simulink model "fft01c"  (R2023a)
settings: Solver=VariableStepAuto  StartTime=0.0  StopTime=10.0  RelTol=1e-3
libraries: dspsrcs4 x3, dspxfrm3 x2
settings Model: Creator=2361266  LastModifiedBy=2361266

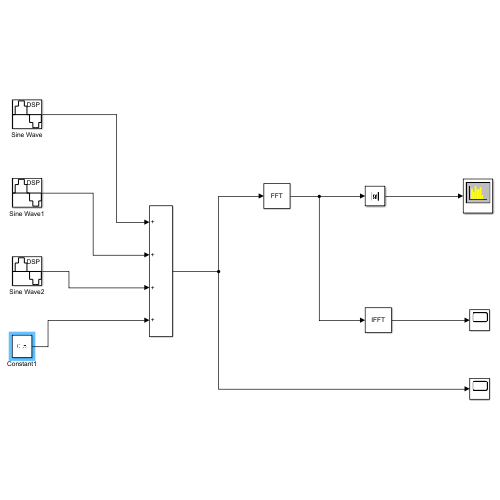
[thumbnail: Simulink's stored preview of the top-level diagram]
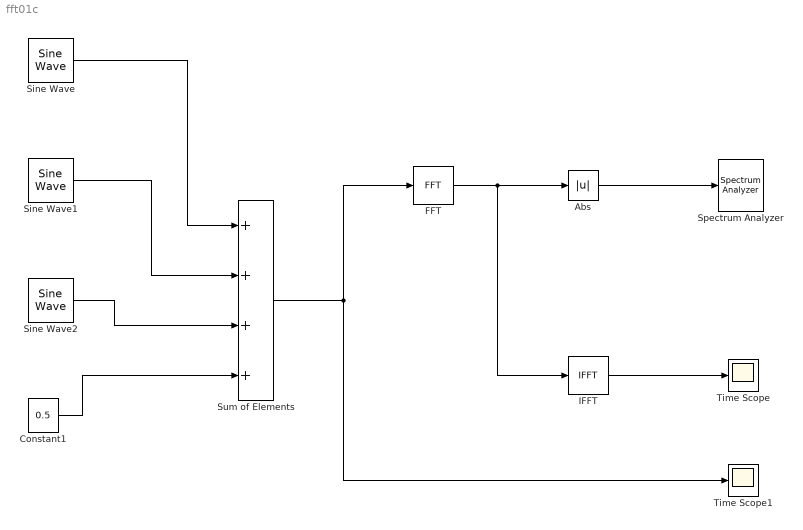
== system fft01c ==
  Abs : Abs  SaturateOnIntegerOverflow=off
  Constant1 : Constant  Value=0.5  VectorParams1D=off
  FFT : dspxfrm3/FFT  FFTImplementation=Auto  CompMethod=Table lookup  TableOpt=NEW  TableOptActive=Speed  BitRevOrder=off  Normalize=off  InheritFFTLength=off  FFTLength=1024  WrapInput=on  roundingMode=Floor  overflowMode=off  firstCoeffDataTypeStr=Inherit: Same word length as input  firstCoeffLastDataTypeStr=Inherit: Same word length as input  outputMin=[]  outputMax=[]
  IFFT : dspxfrm3/IFFT  FFTImplementation=Auto  CompMethod=Table lookup  TableOpt=NEW  TableOptActive=Speed  BitRevOrder=off  cs_in=off  Normalize=off  InheritFFTLength=off  FFTLength=1024  WrapInput=on  mode=Complex  outSamplingMode=Sample based  roundingMode=Floor  overflowMode=off  firstCoeffDataTypeStr=Inherit: Same word length as input  firstCoeffLastDataTypeStr=Inherit: Same word length as input  outputMin=[]  outputMax=[]
  Sine Wave : dspsrcs4/Sine Wave  Amplitude=-4/(pi*pi)  Frequency=50  Phase=pi/2  SampleMode=Discrete  OutComplex=Real  CompMethod=Trigonometric fcn  TableSize=Speed  SampleTime=1/3200  SamplesPerFrame=1024  ResetState=Restart at time zero  OutputFrames=off  dataType=double  wordLen=16  udDataType=sfix(16)  fracBitsMode=Best precision  numFracBits=15  OutDataTypeStr=double  LastOutDataTypeStr=double
  Sine Wave1 : dspsrcs4/Sine Wave  Amplitude=-4/(9*pi*pi)  Frequency=150  Phase=pi/2  SampleMode=Discrete  OutComplex=Real  CompMethod=Trigonometric fcn  TableSize=Speed  SampleTime=1/3200  SamplesPerFrame=1024  ResetState=Restart at time zero  OutputFrames=off  dataType=double  wordLen=16  udDataType=sfix(16)  fracBitsMode=Best precision  numFracBits=15  OutDataTypeStr=double  LastOutDataTypeStr=double
  Sine Wave2 : dspsrcs4/Sine Wave  Amplitude=1/(25*pi*pi)  Frequency=250  Phase=pi/2  SampleMode=Discrete  OutComplex=Real  CompMethod=Trigonometric fcn  TableSize=Speed  SampleTime=1/3200  SamplesPerFrame=1024  ResetState=Restart at time zero  OutputFrames=off  dataType=double  wordLen=16  udDataType=sfix(16)  fracBitsMode=Best precision  numFracBits=15  OutDataTypeStr=double  LastOutDataTypeStr=double
  Spectrum Analyzer : SpectrumAnalyzer  WindowPosition=[570.000000,539.000000,1344.000000,500.000000,]  Visible=on  ScopeFrameLocation=window  FilterSharpness=0.5  YLimits=[0.8989,32.6137]  ColorLimits=[-80 20]  SelectedToolstripTab=spectrumAnalyzerToolstrip.estimationTab
  Sum of Elements : Sum  Inputs=++++
  Time Scope : Scope
  Time Scope1 : Scope
  wires:
  Sine Wave2/1 -> Sum of Elements/3
  Constant1/1 -> Sum of Elements/4
  Sine Wave1/1 -> Sum of Elements/2
  Sine Wave/1 -> Sum of Elements/1
  Sum of Elements/1 -> Time Scope1/1, FFT/1
  FFT/1 -> IFFT/1, Abs/1
  Abs/1 -> Spectrum Analyzer/1
  IFFT/1 -> Time Scope/1
